simulink subsystem "PvtSubSys_PLAN_AP"  (R2020b)
settings: Solver=VariableStepAuto  StartTime=0.0  StopTime=10.0  RelTol=1e-3
undefined symbols (not defined in the file or in its folder): C_LongCtrl_0_Single, C_LongCtrl_0_Uint8, C_LongCtrl_Mph2Kph, magnitude, P_LongCtrl_accelTargAbsThrd, P_LongCtrl_AddVelAccelChange, P_LongCtrl_AddVelAccelThrd, P_LongCtrl_AddVelDistDesThrd, P_LongCtrl_AddVelEnable, P_LongCtrl_AddVelRefMsThrd, P_LongCtrl_ALaLowerChar, P_LongCtrl_ALaUpperCharEco, P_LongCtrl_ALaUpperCharNormal, P_LongCtrl_ALaUpperCharSport, P_LongCtrl_ALCAccLimitByDangerXAxis, P_LongCtrl_ALCAccLimitByDangerYAxis, P_LongCtrl_ALvAcceleLowerChar, P_LongCtrl_ALvAcceleUpperCharEco, P_LongCtrl_ALvAcceleUpperCharNormal, P_LongCtrl_ALvAcceleUpperCharSport, P_LongCtrl_CCaccelCCNeg2PosJerk, P_LongCtrl_CCaccelCCPosJerk, P_LongCtrl_CCaccelLowerIsLaneChange, P_LongCtrl_CCaccelMaxLCActive, P_LongCtrl_CCaccelMinECOAL, P_LongCtrl_CCaccelMinFastDecel, P_LongCtrl_CCaccelMinNoFastDecel, P_LongCtrl_CCaccelMinNormAL, P_LongCtrl_CCaccelMinSportAL, P_LongCtrl_CCaccelUpperCC, P_LongCtrl_CCaccelUpperCCSafeStop, P_LongCtrl_CCaMinNegAcceleLowerBand, P_LongCtrl_CCaMinNegAcceleUpperBand, P_LongCtrl_CCaMinPosAcceleLowerBand, P_LongCtrl_CCaMinPosAcceleUpperBand, P_LongCtrl_CCbECO, P_LongCtrl_CCbNorm, P_LongCtrl_CCbSport, P_LongCtrl_CCcoefESPSpd2IPSpd1, P_LongCtrl_CCcoefESPSpd2IPSpd2, P_LongCtrl_CCdecelCCJerk, P_LongCtrl_CCdecelCCJerkNegVLCInternalAcc, P_LongCtrl_CCfacNegAcceleLowerBand, P_LongCtrl_CCfacNegAcceleUpperBand, P_LongCtrl_CCfacPosAcceleLowerBand, P_LongCtrl_CCfacPosAcceleUpperBand, P_LongCtrl_CCkECO, P_LongCtrl_CCkNorm, P_LongCtrl_CCkSport, P_LongCtrl_CCLCIncSetSpdAdd, P_LongCtrl_CCLCIncSetSpdAddCntStartValue, P_LongCtrl_CCResumeDelayDeltaVel, P_LongCtrl_CCtAcceleTimeNeg, P_LongCtrl_CCtAcceleTimeNegCorrXAxis, P_LongCtrl_CCtAcceleTimeNegCorrYAxis, P_LongCtrl_CCtAcceleTimePos, P_LongCtrl_CCtAcceleTimePosCorrXAxis, P_LongCtrl_CCtAcceleTimePosCorrYAxis, P_LongCtrl_CCtStepVelPlan, P_LongCtrl_CCtTotVelPlan ... (+150)
libraries: simulink x62, TrueDurationTime x1
(part 4 of 7)

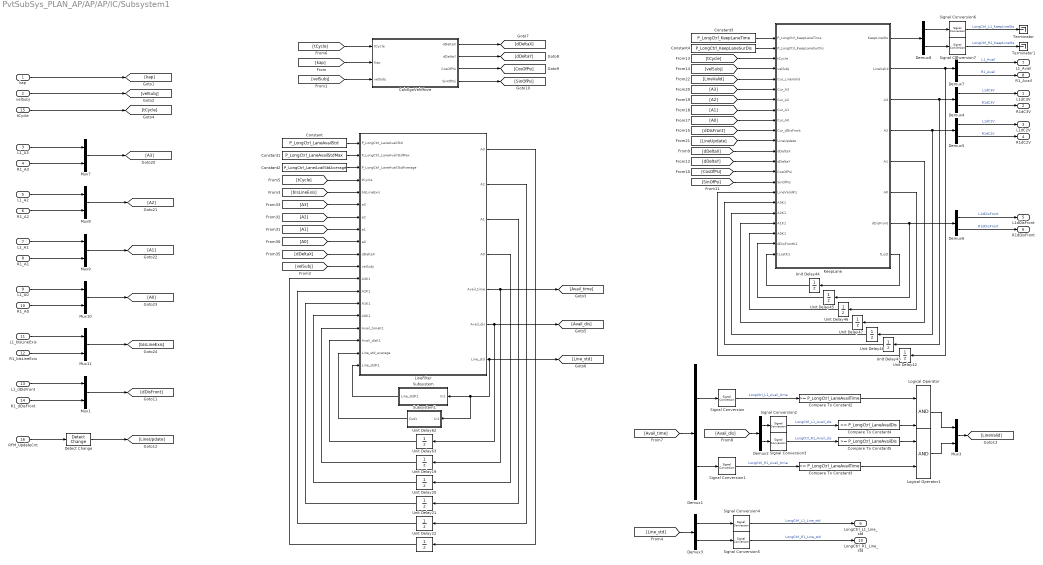
== system PvtSubSys_PLAN_AP/AP/AP/IC/Subsystem1 ==
  kap : Inport
  velSubj : Inport  Port=2
  L1_A3 : Inport  Port=3
  R1_A3 : Inport  Port=4
  L1_A2 : Inport  Port=5
  R1_A2 : Inport  Port=6
  L1_A1 : Inport  Port=7
  R1_A1 : Inport  Port=8
  L1_A0 : Inport  Port=9
  R1_A0 : Inport  Port=10
  L1_bIsLineExis : Inport  Port=11
  R1_bIsLineExis : Inport  Port=12
  L1_dDisFront : Inport  Port=13
  R1_dDisFront : Inport  Port=14
  tCycle : Inport  Port=15
  RFM_UpdateCnt : Inport  Port=16
  CalcEgoVehMove : MATLAB Function  TreatAsAtomicUnit=on
  Compare To Constant2 : simulink/Logic and Bit Operations/Compare To Constant  relop=>=  const=P_LongCtrl_LaneAvailTime  OutDataTypeStr=boolean
  Compare To Constant3 : simulink/Logic and Bit Operations/Compare To Constant  relop=>=  const=P_LongCtrl_LaneAvailTime  OutDataTypeStr=boolean
  Compare To Constant4 : simulink/Logic and Bit Operations/Compare To Constant  relop=>=  const=P_LongCtrl_LaneAvailDis  OutDataTypeStr=boolean
  Compare To Constant5 : simulink/Logic and Bit Operations/Compare To Constant  relop=>=  const=P_LongCtrl_LaneAvailDis  OutDataTypeStr=boolean
  Constant : Constant  Value=P_LongCtrl_LaneAvailStd
  Constant1 : Constant  Value=P_LongCtrl_LaneAvailStdMax
  Constant2 : Constant  Value=P_LongCtrl_LaneAvailStdAverage
  Constant3 : Constant  Value=P_LongCtrl_KeepLaneTime
  Constant4 : Constant  Value=P_LongCtrl_KeepLaneSurDis
  Demux{1..8} (8 alike) : Demux  Outputs=2
  Detect Change : simulink/Logic and Bit Operations/Detect Change  vinit=0  OutDataTypeStr=boolean
  KeepLane : MATLAB Function  TreatAsAtomicUnit=on
  LineFilter : MATLAB Function  TreatAsAtomicUnit=on
  Logical Operator : Logic  AllPortsSameDT=off  OutDataTypeStr=boolean
  Logical Operator1 : Logic  AllPortsSameDT=off  OutDataTypeStr=boolean
  Mux{1,3,7..11} (7 alike) : Mux  Inputs=2
  Signal Conversion{,1..7} (8 alike) : SignalConversion  OverrideOpt=off
  Subsystem : Subsystem
  Subsystem1 : Subsystem
  Terminator : Terminator
  Terminator1 : Terminator
  Unit Delay{19..22} (4 alike) : UnitDelay  InitialCondition=single(zeros(2,1))  SampleTime=-1  HasFrameUpgradeWarning=on
  Unit Delay42 : UnitDelay  InitialCondition=false  SampleTime=-1  HasFrameUpgradeWarning=on
  Unit Delay{43..48} (6 alike) : UnitDelay  InitialCondition=single(0)  SampleTime=-1  HasFrameUpgradeWarning=on
  Unit Delay62 : UnitDelay  InitialCondition=zeros(2,1)  SampleTime=-1  HasFrameUpgradeWarning=on
  Unit Delay63 : UnitDelay  InitialCondition=zeros(2,1)  SampleTime=-1  HasFrameUpgradeWarning=on
  L1dC3V : Outport
  R1dC3V : Outport  Port=2
  L1dC2V : Outport  Port=3
  R1dC2V : Outport  Port=4
  L1dDisFront : Outport  Port=5
  R1dDisFront : Outport  Port=6
  L1_Avail : Outport  Port=7
  R1_Avail : Outport  Port=8
  LongCtrl_L1_Line_std : Outport  Port=9
  LongCtrl_R1_Line_std : Outport  Port=10
  wires:
  Detect Change/1 -> [LineUpdate]
  [tCycle] -> CalcEgoVehMove/1(tCycle)
  [tCycle] -> LineFilter/4(tCycle)
  tCycle/1 -> [tCycle]
  [kap] -> CalcEgoVehMove/2(Kap)
  [velSubj] -> LineFilter/11(velSubj)
  Mux8/1 -> [A2]
  L1_bIsLineExis/1 -> Mux11/1
  L1_A1/1 -> Mux9/1
  kap/1 -> [kap]
  R1_bIsLineExis/1 -> Mux11/2
  Mux10/1 -> [A0]
  LineFilter/5(Avail_time) -> [Avail_time], Unit Delay63/1
  Mux7/1 -> [A3]
  L1_A2/1 -> Mux8/1
  Unit Delay19/1 -> LineFilter/15(A0K1)
  [A2] -> LineFilter/7(a2)
  Unit Delay22/1 -> LineFilter/12(A3K1)
  LineFilter/6(Avail_dis) -> [Avail_dis], Unit Delay62/1
  velSubj/1 -> [velSubj]
  [A1] -> LineFilter/8(a1)
  L1_A3/1 -> Mux7/1
  R1_A0/1 -> Mux10/2
  R1_A2/1 -> Mux8/2
  R1_A1/1 -> Mux9/2
  LineFilter/1(A3) -> Unit Delay22/1
  Unit Delay62/1 -> LineFilter/17(Avail_disK1)
  LineFilter/2(A2) -> Unit Delay21/1
  Mux9/1 -> [A1]
  [A0] -> LineFilter/9(a0)
  LineFilter/4(A0) -> Unit Delay19/1
  R1_A3/1 -> Mux7/2
  Mux11/1 -> [bIsLineExis]
  [bIsLineExis] -> LineFilter/5(bIsLineExis)
  [dDeltaX] -> LineFilter/10(dDeltaX)
  [velSubj] -> CalcEgoVehMove/3(velSubj)
  [A3] -> LineFilter/6(a3)
  LineFilter/3(A1) -> Unit Delay20/1
  Unit Delay20/1 -> LineFilter/14(A1K1)
  L1_A0/1 -> Mux10/1
  Unit Delay63/1 -> LineFilter/16(Avail_timeK1)
  Unit Delay21/1 -> LineFilter/13(A2K1)
  Compare To Constant3/1 -> Logical Operator1/2
  Logical Operator1/1 -> Mux3/2
  Signal Conversion1/1 -> Compare To Constant3/1  "LongCtrl_R1_Avail_time"
  Signal Conversion2/1 -> Compare To Constant4/1  "LongCtrl_L1_Avail_dis"
  Compare To Constant5/1 -> Logical Operator1/1
  Compare To Constant4/1 -> Logical Operator/2
  Logical Operator/1 -> Mux3/1
  Compare To Constant2/1 -> Logical Operator/1
  Signal Conversion3/1 -> Compare To Constant5/1  "LongCtrl_R1_Avail_dis"
  [Avail_time] -> Demux1/1
  Demux2/1 -> Signal Conversion2/1
  [Avail_dis] -> Demux2/1
  Demux2/2 -> Signal Conversion3/1
  Demux1/2 -> Signal Conversion1/1
  Demux1/1 -> Signal Conversion/1
  Signal Conversion/1 -> Compare To Constant2/1  "LongCtrl_L1_Avail_time"
  Constant/1 -> LineFilter/1(P_LongCtrl_LaneAvailStd)
  [Line_std] -> Demux3/1
  Signal Conversion5/1 -> LongCtrl_R1_Line_std/1  "LongCtrl_R1_Line_std"
  Signal Conversion4/1 -> LongCtrl_L1_Line_std/1  "LongCtrl_L1_Line_std"
  Demux3/1 -> Signal Conversion4/1
  Demux3/2 -> Signal Conversion5/1
  LineFilter/7(Line_std) -> [Line_std], Subsystem1/1(In1), Subsystem/1(In1)
  Subsystem/1(Line_stdK1) -> LineFilter/19(Line_stdK1)
  Subsystem1/1(Out1) -> LineFilter/18(Line_std_average)
  CalcEgoVehMove/1(dDeltaX) -> [dDeltaX]
  CalcEgoVehMove/2(dDeltaY) -> [dDeltaY]
  CalcEgoVehMove/4(SinOfPsi) -> [SinOfPsi]
  CalcEgoVehMove/3(CosOfPsi) -> [CosOfPsi]
  KeepLane/8(tLost) -> Unit Delay44/1
  Unit Delay42/1 -> KeepLane/16(LineValidK1)
  [CosOfPsi] -> KeepLane/14(CosOfPsi)
  [dDeltaY] -> KeepLane/13(dDeltaY)
  [dDeltaX] -> KeepLane/12(dDeltaX)
  Unit Delay43/1 -> KeepLane/17(A3K1)
  [SinOfPsi] -> KeepLane/15(SinOfPsi)
  Unit Delay48/1 -> KeepLane/18(A2K1)
  KeepLane/5(A1) -> Unit Delay47/1
  KeepLane/3(A3) -> Demux4/1, Unit Delay43/1
  Unit Delay46/1 -> KeepLane/20(A0K1)
  Unit Delay45/1 -> KeepLane/21(dDisFrontK1)
  Unit Delay44/1 -> KeepLane/22(tLostK1)
  KeepLane/2(LineValid) -> Demux7/1, Unit Delay42/1
  KeepLane/4(A2) -> Demux5/1, Unit Delay48/1
  KeepLane/6(A0) -> Unit Delay46/1
  Unit Delay47/1 -> KeepLane/19(A1K1)
  Mux1/1 -> [dDisFront]
  R1_dDisFront/1 -> Mux1/2
  L1_dDisFront/1 -> Mux1/1
  RFM_UpdateCnt/1 -> Detect Change/1
  Mux3/1 -> [LineValid]
  Constant1/1 -> LineFilter/2(P_LongCtrl_LaneAvailStdMax)
  Constant2/1 -> LineFilter/3(P_LongCtrl_LaneAvailStdAverage)
  [tCycle] -> KeepLane/3(tCycle)
  [velSubj] -> KeepLane/4(velSubj)
  [LineValid] -> KeepLane/5(Cur_LineValid)
  [A3] -> KeepLane/6(Cur_A3)
  [A2] -> KeepLane/7(Cur_A2)
  [A1] -> KeepLane/8(Cur_A1)
  [A0] -> KeepLane/9(Cur_A0)
  [dDisFront] -> KeepLane/10(Cur_dDisFront)
  [LineUpdate] -> KeepLane/11(LineUpdate)
  Constant3/1 -> KeepLane/1(P_LongCtrl_KeepLaneTime)
  Constant4/1 -> KeepLane/2(P_LongCtrl_KeepLaneSurDis)
  Demux4/1 -> L1dC3V/1  "L1dC3V"
  Demux4/2 -> R1dC3V/1  "R1dC3V"
  Demux5/2 -> R1dC2V/1  "R1dC2V"
  Demux5/1 -> L1dC2V/1  "L1dC2V"
  Demux6/1 -> L1dDisFront/1  "L1dDisFront"
  Demux6/2 -> R1dDisFront/1  "R1dDisFront"
  KeepLane/7(dDisFront) -> Unit Delay45/1, Demux6/1
  Demux7/2 -> R1_Avail/1  "R1_Avail"
  Demux7/1 -> L1_Avail/1  "L1_Avail"
  KeepLane/1(KeepLineSts) -> Demux8/1
  Demux8/1 -> Signal Conversion6/1
  Demux8/2 -> Signal Conversion7/1
  Signal Conversion6/1 -> Terminator/1  "LongCtrl_L1_KeepLineSts"
  Signal Conversion7/1 -> Terminator1/1  "LongCtrl_R1_KeepLineSts"

== system PvtSubSys_PLAN_AP/AP/AP/ORD/BandJerkCalc ==
  accelOffRamp : Inport
  Add : Sum
  Add1 : Sum  Inputs=+-
  Constant : Constant  Value=P_LongCtrl_ORDaccelDevUpperBand  OutDataTypeStr=single
  Constant1 : Constant  Value=P_LongCtrl_ORDaccelDevLowerBand  OutDataTypeStr=single
  Constant2 : Constant  Value=P_LongCtrl_ORDupperJerk  OutDataTypeStr=single
  Constant3 : Constant  Value=P_LongCtrl_ORDlowerJerk  OutDataTypeStr=single
  upperBandORD : Outport
  lowerBandORD : Outport  Port=2
  upperJerkORD : Outport  Port=3
  lowerJerkORD : Outport  Port=4
  wires:
  accelOffRamp/1 -> Add/1, Add1/1
  Constant/1 -> Add/2
  Constant1/1 -> Add1/2
  Add/1 -> upperBandORD/1  "upperBandORD"
  Add1/1 -> lowerBandORD/1  "lowerBandORD"
  Constant2/1 -> upperJerkORD/1  "upperJerkORD"
  Constant3/1 -> lowerJerkORD/1  "lowerJerkORD"

== system PvtSubSys_PLAN_AP/AP/AP/ORD/ORD/accelOffRampDistExceed ==
  distRamp2Cur : Inport  OutDataTypeStr=uint16  PortDimensions=1
  StartVel : Inport  Port=2  OutDataTypeStr=single  PortDimensions=1
  EndVel : Inport  Port=3  OutDataTypeStr=uint8  PortDimensions=1
  f : TriggerPort  TriggerType=function-call  VariantControl=(inherit)
      settings: CopyFcn=Stateflow.SLINSF.SimulinkMan.removeBlockPreDeleteFcn  PreDeleteFcn=Stateflow.SLINSF.SimulinkMan.unsafePredeleteFcn
  Add : Sum  Inputs=-+
  Constant : Constant  Value=2  OutDataTypeStr=single
  Constant2 : Constant  Value=10  OutDataTypeStr=single
  Constant3 : Constant  Value=3.6  OutDataTypeStr=single
  Constant4 : Constant  Value=3.6  OutDataTypeStr=single
  MinMax : MinMax  Function=max  Inputs=2
  Product : Product
  Product1 : Product  Inputs=*/
  Product3 : Product
  Product4 : Product
  Product5 : Product  Inputs=*/
  Product6 : Product  Inputs=*/
  accelOffRamp : Outport
  wires:
  Product4/1 -> Add/2
  Product3/1 -> Add/1
  Product6/1 -> Product4/1, Product4/2
  EndVel/1 -> Product6/1
  Constant4/1 -> Product6/2
  Constant3/1 -> Product5/2
  Product5/1 -> Product3/1, Product3/2
  StartVel/1 -> Product5/1
  distRamp2Cur/1 -> MinMax/1
  Constant/1 -> Product/2
  Add/1 -> Product1/1
  Product/1 -> Product1/2
  Product1/1 -> accelOffRamp/1  "accelOffRamp"
  Constant2/1 -> MinMax/2
  MinMax/1 -> Product/1

== system PvtSubSys_PLAN_AP/AP/AP/ORD/ORD/accelOffRampNegCalc ==
  velDelta : Inport  OutDataTypeStr=single  PortDimensions=1
  f : TriggerPort  TriggerType=function-call  VariantControl=(inherit)
      settings: CopyFcn=Stateflow.SLINSF.SimulinkMan.removeBlockPreDeleteFcn  PreDeleteFcn=Stateflow.SLINSF.SimulinkMan.unsafePredeleteFcn
  Constant : Constant  Value=P_LongCtrl_ORDtAcceleTimeNeg  OutDataTypeStr=single
  Product : Product  Inputs=*/
  accelOffRamp : Outport
  wires:
  velDelta/1 -> Product/1
  Constant/1 -> Product/2
  Product/1 -> accelOffRamp/1  "accelOffRamp"

== system PvtSubSys_PLAN_AP/AP/AP/ORD/ORD/accelOffRampPosCalc ==
  velDelta : Inport  OutDataTypeStr=single  PortDimensions=1
  f : TriggerPort  TriggerType=function-call  VariantControl=(inherit)
      settings: CopyFcn=Stateflow.SLINSF.SimulinkMan.removeBlockPreDeleteFcn  PreDeleteFcn=Stateflow.SLINSF.SimulinkMan.unsafePredeleteFcn
  Constant : Constant  Value=P_LongCtrl_ORDtAcceleTimePos  OutDataTypeStr=single
  Product : Product  Inputs=*/
  accelOffRamp : Outport
  wires:
  velDelta/1 -> Product/1
  Constant/1 -> Product/2
  Product/1 -> accelOffRamp/1  "accelOffRamp"

== system PvtSubSys_PLAN_AP/AP/AP/ORD/ORD/distDesOffRampCalc ==
  StartVel : Inport  OutDataTypeStr=single  PortDimensions=1
  EndVel : Inport  Port=2  OutDataTypeStr=uint8  PortDimensions=1
  accelOffRamp : Inport  Port=3  OutDataTypeStr=single  PortDimensions=1
  f : TriggerPort  TriggerType=function-call  VariantControl=(inherit)
      settings: CopyFcn=Stateflow.SLINSF.SimulinkMan.removeBlockPreDeleteFcn  PreDeleteFcn=Stateflow.SLINSF.SimulinkMan.unsafePredeleteFcn
  Abs : Abs
  Abs1 : Abs
  Add : Sum  Inputs=-+
  Constant : Constant  Value=2  OutDataTypeStr=single
  Constant3 : Constant  Value=3.6  OutDataTypeStr=single
  Constant4 : Constant  Value=3.6  OutDataTypeStr=single
  Product : Product  Inputs=*/
  Product1 : Product
  Product3 : Product
  Product4 : Product
  Product5 : Product  Inputs=*/
  Product6 : Product  Inputs=*/
  distDesOffRamp : Outport
  wires:
  Add/1 -> Abs1/1
  Constant4/1 -> Product6/2
  EndVel/1 -> Product6/1
  Product5/1 -> Product3/1, Product3/2
  StartVel/1 -> Product5/1
  Product6/1 -> Product4/1, Product4/2
  Product4/1 -> Add/2
  Constant3/1 -> Product5/2
  Product3/1 -> Add/1
  Abs1/1 -> Product/1
  accelOffRamp/1 -> Abs/1
  Constant/1 -> Product1/2
  Product1/1 -> Product/2
  Product/1 -> distDesOffRamp/1  "distDesOffRamp"
  Abs/1 -> Product1/1

== system PvtSubSys_PLAN_AP/AP/AP/ORD/ORD/velDeltaCalc ==
  velOffRampLimit : Inport  OutDataTypeStr=uint8  PortDimensions=1
  vehicleSpd : Inport  Port=2  OutDataTypeStr=single  PortDimensions=1
  f : TriggerPort  TriggerType=function-call  VariantControl=(inherit)
      settings: CopyFcn=Stateflow.SLINSF.SimulinkMan.removeBlockPreDeleteFcn  PreDeleteFcn=Stateflow.SLINSF.SimulinkMan.unsafePredeleteFcn
  Add : Sum  Inputs=+-
  Add1 : Sum
  Constant : Constant  Value=1.03  OutDataTypeStr=single
  Constant1 : Constant  Value=1.3  OutDataTypeStr=single
  Constant2 : Constant  Value=3.6  OutDataTypeStr=single
  Product : Product
  Product1 : Product  Inputs=*/
  velDelta : Outport
  IPKVel : Outport  Port=2
  wires:
  velOffRampLimit/1 -> Add/1
  vehicleSpd/1 -> Product/1
  Constant/1 -> Product/2
  Product/1 -> Add1/1
  Constant1/1 -> Add1/2
  Add1/1 -> Add/2, IPKVel/1
  Add/1 -> Product1/1
  Constant2/1 -> Product1/2
  Product1/1 -> velDelta/1  "velDelta"

== system PvtSubSys_PLAN_AP/AP/AP/SJ/BrakePreferJudge ==
  TargetExistP0 : Inport
  accelFollow : Inport  Port=2
  accelSubjPlanOpt : Inport  Port=3
  VlcInternalAccK1 : Inport  Port=4
  axvRoadSlopeMs2 : Inport  Port=5
  accelSubj : Inport  Port=6
  ttc : Inport  Port=7
  ACCModeSts : Inport  Port=8
  velSubj : Inport  Port=9
  HWASlowQuit : Inport  Port=10
  Compare To Constant : simulink/Logic and Bit Operations/Compare To Constant  relop===  const=1  OutDataTypeStr=boolean
  Compare To Constant1 : simulink/Logic and Bit Operations/Compare To Constant  relop=<  const=P_LongCtrl_SJaccelFollowThresEnableBrkPrefer  OutDataTypeStr=boolean
  Compare To Constant2 : simulink/Logic and Bit Operations/Compare To Constant  relop=<  const=P_LongCtrl_SJaccelSubjPlanOptThresEnableBrkPrefer  OutDataTypeStr=boolean
  Compare To Constant3 : simulink/Logic and Bit Operations/Compare To Constant  relop=<  const=P_LongCtrl_SJVlcInternalAccThresEnableBrkPrefer  OutDataTypeStr=boolean
  Compare To Constant4 : simulink/Logic and Bit Operations/Compare To Constant  relop=<  const=P_LongCtrl_SJaxvRoadSlopeThresEnableBrkPrefer  OutDataTypeStr=boolean
  Compare To Constant5 : simulink/Logic and Bit Operations/Compare To Constant  relop=>  const=P_LongCtrl_SJaccelSubjThresEnableBrkPrefer  OutDataTypeStr=boolean
  Compare To Constant6 : simulink/Logic and Bit Operations/Compare To Constant  relop=<  const=P_LongCtrl_SJttcThresEnableBrkPrefer  OutDataTypeStr=boolean
  Compare To Constant7 : simulink/Logic and Bit Operations/Compare To Constant  relop===  const=3  OutDataTypeStr=boolean
  Compare To Constant8 : simulink/Logic and Bit Operations/Compare To Constant  relop=>  const=P_LongCtrl_SJvelSubjThresEnableBrkPrefer  OutDataTypeStr=boolean
  Logical Operator : Logic  Inputs=9  AllPortsSameDT=off  OutDataTypeStr=boolean
  Logical Operator1 : Logic  Operator=OR  AllPortsSameDT=off  OutDataTypeStr=boolean
  MinMax : MinMax
  BrakePrefer : Outport
  wires:
  Logical Operator1/1 -> BrakePrefer/1  "BrakePrefer"
  TargetExistP0/1 -> Compare To Constant/1  "TargetExistP0"
  accelFollow/1 -> Compare To Constant1/1  "accelFollow"
  accelSubjPlanOpt/1 -> MinMax/1  "accelSubjPlanOpt"
  VlcInternalAccK1/1 -> Compare To Constant3/1  "VlcInternalAccK1"
  axvRoadSlopeMs2/1 -> Compare To Constant4/1  "axvRoadSlopeMs2"
  accelSubj/1 -> Compare To Constant5/1  "accelSubj"
  ttc/1 -> Compare To Constant6/1  "ttc"
  MinMax/1 -> Compare To Constant2/1
  ACCModeSts/1 -> Compare To Constant7/1  "ACCModeSts"
  Compare To Constant/1 -> Logical Operator/2
  Compare To Constant1/1 -> Logical Operator/3
  Compare To Constant2/1 -> Logical Operator/4
  Compare To Constant3/1 -> Logical Operator/5
  Compare To Constant4/1 -> Logical Operator/6
  Compare To Constant5/1 -> Logical Operator/7
  Compare To Constant7/1 -> Logical Operator/1
  Compare To Constant6/1 -> Logical Operator/8
  velSubj/1 -> Compare To Constant8/1  "velSubj"
  Compare To Constant8/1 -> Logical Operator/9
  Logical Operator/1 -> Logical Operator1/1  "BrakePrefer"
  HWASlowQuit/1 -> Logical Operator1/2  "HWASlowQuit"

== system PvtSubSys_PLAN_AP/AP/AP/SJ/DeceleToStop ==
  DriveOffConditonFulfilled : Inport
  TargetExistP0 : Inport  Port=2
  ACCModeSts : Inport  Port=3
  velSubj : Inport  Port=4
  velTargetRel : Inport  Port=5
  VlcInternalAcc : Inport  Port=6
  distTargRel : Inport  Port=7
  SafeStopActive : Inport  Port=8
  axvRoadSlopeMs2 : Inport  Port=9
  1-D Lookup Table : Lookup_n-D  NumberOfTableDimensions=1  BreakpointsForDimension1=P_LongCtrl_distThreDecToStopXAxis  Table=P_LongCtrl_distThreDecToStopYAxis  ExtrapMethod=Clip  InternalRulePriority=Speed  RndMeth=Simplest  InputSameDT=on
  DeceleToStop : Stateflow chart  TreatAsAtomicUnit=on
  DecleToStop : Outport
  wires:
  SafeStopActive/1 -> DeceleToStop/8(SafeStopActive)  "SafeStopActive"
  DriveOffConditonFulfilled/1 -> DeceleToStop/7(DriveOffConditonFulfilled)  "DriveOffConditonFulfilled"
  DeceleToStop/1(DecleToStop) -> DecleToStop/1  "DecleToStop"
  VlcInternalAcc/1 -> DeceleToStop/5(VlcInternalAcc)  "VlcInternalAcc"
  distTargRel/1 -> DeceleToStop/6(distTargRel)  "distTargRel"
  ACCModeSts/1 -> DeceleToStop/4(ACCModeSts)  "ACCModeSts"
  TargetExistP0/1 -> DeceleToStop/3(TargetExistP0)  "TargetExistP0"
  velTargetRel/1 -> DeceleToStop/2(velTargetRel)  "velTargetRel"
  velSubj/1 -> DeceleToStop/1(velSubj)  "velSubj"
  axvRoadSlopeMs2/1 -> 1-D Lookup Table/1  "axvRoadSlopeMs2"
  1-D Lookup Table/1 -> DeceleToStop/9(distThreDecToStop)

== system PvtSubSys_PLAN_AP/AP/AP/SJ/DisBar ==
  distTargRel : Inport
  DesireDistanceChar : Inport  Port=2
  timeGapSet : Inport  Port=3
  ACCSts_ACCModeSts : Inport  Port=4
  P0_Exist : Inport  Port=5
  distTargRelP2 : Inport  Port=6
  distTargRelP3 : Inport  Port=7
  P2_Exist : Inport  Port=8
  P3_Exist : Inport  Port=9
  ACC_DisplayBar1 : Subsystem  TreatAsAtomicUnit=on
  Constant18 : Constant  Value=[0.6,0.75,0.9;0.58,0.68,0.77;0.41,0.55,0.63;0.38,0.44,0.49]  OutDataTypeStr=single
  Demux : Demux  Outputs=3
  Mux2 : Mux  Inputs=3
  Mux3 : Mux  Inputs=3
  Signal Conversion : SignalConversion  OverrideOpt=off
  Signal Conversion1 : SignalConversion  OverrideOpt=off
  Signal Conversion2 : SignalConversion  OverrideOpt=off
  ACC_TgtObjBarDisp : Outport  OutDataTypeStr=uint8
  ACC_LeTgtObjBarDisp : Outport  Port=2
  ACC_RiTgtObjBarDisp : Outport  Port=3
  wires:
  Signal Conversion2/1 -> ACC_RiTgtObjBarDisp/1
  Signal Conversion1/1 -> ACC_LeTgtObjBarDisp/1
  Signal Conversion/1 -> ACC_TgtObjBarDisp/1
  P3_Exist/1 -> Mux3/3
  P0_Exist/1 -> Mux3/1
  distTargRelP2/1 -> Mux2/2
  Constant18/1 -> ACC_DisplayBar1/5(Scale)
  distTargRelP3/1 -> Mux2/3
  Mux2/1 -> ACC_DisplayBar1/4(TargetRange)
  P2_Exist/1 -> Mux3/2
  Mux3/1 -> ACC_DisplayBar1/6(TargetExist)
  ACC_DisplayBar1/1(Signal_ACC_TgtObjBarDisp) -> Demux/1  "ACC_TgtObjBarDisp"
  Demux/2 -> Signal Conversion1/1  "ACC_LeTgtObjBarDisp"
  Demux/1 -> Signal Conversion/1  "ACC_TgtObjBarDisp"
  Demux/3 -> Signal Conversion2/1  "ACC_RiTgtObjBarDisp"
  distTargRel/1 -> Mux2/1  "distTargRel"
  timeGapSet/1 -> ACC_DisplayBar1/1(TimeGap)  "timeGapSet"
  DesireDistanceChar/1 -> ACC_DisplayBar1/2(DesireDistance)
  ACCSts_ACCModeSts/1 -> ACC_DisplayBar1/3(ACCmode)

== system PvtSubSys_PLAN_AP/AP/AP/SJ/DriverOffConditionFulfilled ==
  TargetExistP0 : Inport
  velTargetRel : Inport  Port=2
  VelSet : Inport  Port=3  OutDataTypeStr=single
  distDesCur : Inport  Port=4
  velSubj : Inport  Port=5
  distTargRel : Inport  Port=6
  safeStopActive : Inport  Port=7
  ACCModeSts : Inport  Port=8
  ObjTypeP0 : Inport  Port=9
  Compare To Constant : simulink/Logic and Bit Operations/Compare To Constant  relop===  const=0  OutDataTypeStr=boolean
  Compare To Constant1 : simulink/Logic and Bit Operations/Compare To Constant  relop=>  const=0  OutDataTypeStr=boolean
  Constant : Constant  Value=0  OutDataTypeStr=uint8
  DriveOff_Judge : Stateflow chart  TreatAsAtomicUnit=on
  Gain : Gain  Gain=1/3.6
  Switch : Switch  Criteria=u2 > Threshold
  DriveOffConditonFulfilled : Outport  OutDataTypeStr=boolean
  wires:
  ObjTypeP0/1 -> DriveOff_Judge/8(ObjTypeP0)
  safeStopActive/1 -> Compare To Constant/1
  Compare To Constant/1 -> Switch/2
  velSubj/1 -> DriveOff_Judge/1(velSubj)  "velSubj"
  VelSet/1 -> Gain/1  "VelSet"
  velTargetRel/1 -> DriveOff_Judge/4(velTargRel)  "velTargetRel"
  distTargRel/1 -> DriveOff_Judge/5(distTargRel)  "distTargRel"
  TargetExistP0/1 -> DriveOff_Judge/6(targetExist)  "TargetExistP0"
  Constant/1 -> Switch/3
  Gain/1 -> DriveOff_Judge/3(velSet)
  Compare To Constant1/1 -> DriveOffConditonFulfilled/1
  ACCModeSts/1 -> DriveOff_Judge/7(ACCModeSts)  "ACCModeSts"
  DriveOff_Judge/1(DriveOffConditonFulfilled) -> Switch/1
  Switch/1 -> Compare To Constant1/1  "DriveOffConditonFulfilled"
  distDesCur/1 -> DriveOff_Judge/2(dDesired)  "distDesCur"

== system PvtSubSys_PLAN_AP/AP/AP/SJ/TakeOver ==
  accelFollow : Inport
  ACCModeSts : Inport  Port=2
  distTargetRel : Inport  Port=3
  velSubj : Inport  Port=4
  targetExistP0 : Inport  Port=5
  distRelPlanMin : Inport  Port=6
  distRelDesDistRelPlanNumMin : Inport  Port=7
  velTargetRel : Inport  Port=8
  tCycle : Inport  Port=9
  Chart : Stateflow chart  TreatAsAtomicUnit=on
      settings: PortSchema="{\"entries\":[{\"content\":{\"sides\":[{\"content\":{\"connectorIds\":[\"In1\",\"In2\",\"In3\"]},\"type\":\"ConnectorPlacement.EquallySpacedRectSide\",\"uuid\":\"a9be611c-1302-4d01-95c8-aa310eaae015\"},{\"content\":{\"connectorIds\":[\"Out2\",\"Out1\"],\"side\":\"RIGHT\"},\"type\":\"ConnectorPlacement.EquallySpacedRectSide\",\"uuid\":\"1ce4f311-da37-41d3-8dab-86903ba1c2a6\"},{\"content\":{\"connectorIds\":[],\"side\":\"TOP\"},\"type\":\"ConnectorPlacement.EquallySpacedRectSide\",\"uuid\":\"6f48286d-1440-4f3e-bf88-8b89e91ed982\"},{\"content\":{\"connectorIds\":[],\"side\":\"HIDDEN\"},\"type\":\"ConnectorPlacement.EquallySpacedRectSide\",\"uuid\":\"bdda7e3f-a505-4bee-9100-0395b80b4afd\"}]},\"type\":\"ConnectorPlacement.EquallySpacedConnector\",\"uuid\":\"e8fe679d-9fc6-4d49-831a-9b3ad6242aaa\"}],\"packageUris\":[\"http://schema.mathworks.com/mf0/Connector/R2020b\"],\"version\":\"1.0\"}"
  Constant : Constant  Value=P_LongCtrl_WaitTime
  Divide : Product  Inputs=*/
  Gap : Subsystem
  TakeOver : Stateflow chart  TreatAsAtomicUnit=on
  Terminator : Terminator
  tor : Outport
  wires:
  ACCModeSts/1 -> TakeOver/1(ACCModeSts)
  accelFollow/1 -> TakeOver/3(accelFollow)
  distTargetRel/1 -> Gap/1(distTargetRel)
  velSubj/1 -> Gap/2(velSubj)
  Gap/1(gap) -> TakeOver/2(gap)
  targetExistP0/1 -> TakeOver/4(targetExistP0)
  distRelPlanMin/1 -> Chart/2(distRelPlanMin)
  distRelDesDistRelPlanNumMin/1 -> Chart/3(distRelDesDistRelPlanNumMin)
  velTargetRel/1 -> TakeOver/5(velTargetRel)
  TakeOver/1(tor) -> tor/1
  Divide/1 -> Chart/1(WaitSteps)
  Constant/1 -> Divide/1
  tCycle/1 -> Divide/2
  Chart/1(Cnt) -> Terminator/1
  Chart/2(TorCtrlReq) -> TakeOver/6(TorCtrlReq)

== system PvtSubSys_PLAN_AP/AP/AP/FollowCtrl/AccelTargFilter/accelTargAbsFilter/tFiltP0Calc ==
  diffAccelCur2K1P0 : Inport  OutDataTypeStr=single  PortDimensions=1
  f : TriggerPort  TriggerType=function-call  VariantControl=Variant
      settings: CopyFcn=Stateflow.SLINSF.SimulinkMan.removeBlockPreDeleteFcn  PreDeleteFcn=Stateflow.SLINSF.SimulinkMan.unsafePredeleteFcn
  1-D Lookup Table : Lookup_n-D  NumberOfTableDimensions=1  BreakpointsForDimension1=P_LongCtrl_FollowTFiltP0XAxis  Table=P_LongCtrl_FollowTFiltP0YAxis  ExtrapMethod=Clip  InternalRulePriority=Speed  RndMeth=Simplest  InputSameDT=on
  tFiltP0 : Outport
  wires:
  1-D Lookup Table/1 -> tFiltP0/1  "tFiltP0"
  diffAccelCur2K1P0/1 -> 1-D Lookup Table/1

== system PvtSubSys_PLAN_AP/AP/AP/FollowCtrl/DecelToStopCtrl/DecelToStopCtrl ==
  note: when runtime is 50ms,this value is -0.025.
  note: when runtime is 20ms,this value is -0.01.
  FollowAccelMPC : Inport
  accelTargAbs : Inport  Port=2
  distTargRel : Inport  Port=3
  velSubj : Inport  Port=4
  distDesCur : Inport  Port=5
  velTargAbs : Inport  Port=6
  ACCModeSts : Inport  Port=7  OutDataTypeStr=uint8
  DrvOFF_Req : Inport  Port=8
  axvRoadSlopeMs2 : Inport  Port=9
  ObjMovingStateP0 : Inport  Port=10
  DecelToStopCtrl : Stateflow chart  TreatAsAtomicUnit=on
      settings: PortSchema="{\"entries\":[{\"content\":{\"sides\":[{\"content\":{\"connectorIds\":[\"In1\",\"In2\",\"In3\",\"In4\",\"In5\",\"In6\",\"In7\",\"In8\",\"In9\",\"In10\",\"In11\",\"In12\",\"In13\",\"In14\",\"In15\",\"In16\",\"In17\",\"In18\",\"In19\",\"In20\",\"In22\",\"In23\",\"In24\",\"In25\",\"In26\",\"In21\"]},\"type\":\"ConnectorPlacement.EquallySpacedRectSide\",\"uuid\":\"c20511a8-015c-4635-8210-b9eed3497188\"},{\"content\":{\"connectorIds\":[\"Out1\",\"Out2\"],\"side\":\"RIGHT\"},\"type\":\"ConnectorPlacement.EquallySpacedRectSide\",\"uuid\":\"1a046c23-c67c-4e6f-902f-f121eb708ec4\"},{\"content\":{\"connectorIds\":[],\"side\":\"TOP\"},\"type\":\"ConnectorPlacement.EquallySpacedRectSide\",\"uuid\":\"c73ac045-3121-4509-a6aa-8453b68f107e\"},{\"content\":{\"connectorIds\":[],\"side\":\"HIDDEN\"},\"type\":\"ConnectorPlacement.EquallySpacedRectSide\",\"uuid\":\"793d462e-a4a7-4165-a400-0e9fce0ddd3d\"}]},\"type\":\"ConnectorPlacement.EquallySpacedConnector\",\"uuid\":\"1cf22de0-f5b0-4ce2-b122-91219d3d6299\"}],\"packageUris\":[\"http://schema.mathworks.com/mf0/Connector/R2020b\"],\"version\":\"1.0\"}"
  P_LongCtrl_AddVelAccelChange : Constant  Value=P_LongCtrl_AddVelAccelChange
  P_LongCtrl_AddVelAccelThrd : Constant  Value=P_LongCtrl_AddVelAccelThrd
  P_LongCtrl_AddVelDistDesThrd : Constant  Value=P_LongCtrl_AddVelDistDesThrd
  P_LongCtrl_AddVelEnable : Constant  Value=P_LongCtrl_AddVelEnable
  P_LongCtrl_AddVelRefMsThrd : Constant  Value=P_LongCtrl_AddVelRefMsThrd
  P_LongCtrl_FollowaccelStopMax : Constant  Value=P_LongCtrl_FollowaccelStopMax  OutDataTypeStr=single
  P_LongCtrl_FollowaccelTargThresEnableStop : Constant  Value=P_LongCtrl_FollowaccelTargThresEnableStop  OutDataTypeStr=single
  P_LongCtrl_FollowaccelTargThresForceStop : Constant  Value=P_LongCtrl_FollowaccelTargThresForceStop  OutDataTypeStr=single
  P_LongCtrl_FollowdistThresEnableStop : Constant  Value=P_LongCtrl_FollowdistThresEnableStop  OutDataTypeStr=single
  P_LongCtrl_FollowvelSubjThresEnableStop : Constant  Value=P_LongCtrl_FollowvelSubjThresEnableStop  OutDataTypeStr=single
  P_LongCtrl_FollowvelTarAbsThresForceStop : Constant  Value=P_LongCtrl_FollowvelTarAbsThresForceStop  OutDataTypeStr=single
  P_LongCtrl_jerkForceStop : Constant  Commented=on  Value=-0.025  OutDataTypeStr=single
  P_LongCtrl_jerkForceStop1 : Constant  Commented=on  Value=-0.01  OutDataTypeStr=single
  P_LongCtrl_velSubjThresEnableStopAdd : Subsystem
  Subsystem : Subsystem
  FollowAccel : Outport
  ForceStop : Outport  Port=2
  wires:
  P_LongCtrl_AddVelAccelChange/1 -> DecelToStopCtrl/26(P_LongCtrl_AddVelAccelChange)
  P_LongCtrl_AddVelEnable/1 -> DecelToStopCtrl/25(P_LongCtrl_AddVelEnable)
  P_LongCtrl_AddVelRefMsThrd/1 -> DecelToStopCtrl/24(P_LongCtrl_AddVelRefMsThrd)
  P_LongCtrl_AddVelDistDesThrd/1 -> DecelToStopCtrl/23(P_LongCtrl_AddVelDistDesThrd)
  P_LongCtrl_AddVelAccelThrd/1 -> DecelToStopCtrl/22(P_LongCtrl_AddVelAccelThrd)
  ObjMovingStateP0/1 -> DecelToStopCtrl/21(ObjMovingStateP0)
  DrvOFF_Req/1 -> DecelToStopCtrl/7(DrvOFF_Req)  "DrvOFF_Req"
  P_LongCtrl_FollowvelTarAbsThresForceStop/1 -> DecelToStopCtrl/20(P_LongCtrl_velTarAbsThresForceStop)
  velTargAbs/1 -> DecelToStopCtrl/5(velTargAbs)
  ACCModeSts/1 -> DecelToStopCtrl/6(ACCModeSts)
  P_LongCtrl_FollowaccelTargThresForceStop/1 -> DecelToStopCtrl/19(P_LongCtrl_accelTargThresForceStop)
  distDesCur/1 -> DecelToStopCtrl/4(distDesCur)
  accelTargAbs/1 -> DecelToStopCtrl/1(accelTargAbs)
  distTargRel/1 -> DecelToStopCtrl/8(distTargRel), P_LongCtrl_velSubjThresEnableStopAdd/1(distTargRel)
  velSubj/1 -> DecelToStopCtrl/2(velSubj)
  FollowAccelMPC/1 -> DecelToStopCtrl/3(FollowAccelDes)
  P_LongCtrl_FollowdistThresEnableStop/1 -> DecelToStopCtrl/15(P_LongCtrl_distThresEnableStop)
  P_LongCtrl_FollowvelSubjThresEnableStop/1 -> DecelToStopCtrl/16(P_LongCtrl_velSubjThresEnableStop)
  P_LongCtrl_FollowaccelTargThresEnableStop/1 -> DecelToStopCtrl/17(P_LongCtrl_accelTargThresEnableStop)
  P_LongCtrl_FollowaccelStopMax/1 -> DecelToStopCtrl/18(P_LongCtrl_accelStopMax)
  DecelToStopCtrl/1(FollowAccel) -> FollowAccel/1
  DecelToStopCtrl/2(ForceStop) -> ForceStop/1  "ForceStop"
  P_LongCtrl_velSubjThresEnableStopAdd/2(velSubjThresEnableStopAdd) -> DecelToStopCtrl/10(velSubjThresEnableStopAdd)
  P_LongCtrl_velSubjThresEnableStopAdd/1(accelFollowDesThresEnableStop) -> DecelToStopCtrl/9(accelFollowDesThresEnableStop)
  axvRoadSlopeMs2/1 -> Subsystem/1(axvRoadSlopeMs2)
  Subsystem/1(velSubjThresForceStop) -> DecelToStopCtrl/12(velSubjThresForceStop), P_LongCtrl_velSubjThresEnableStopAdd/2(velSubjThresForceStop)
  Subsystem/2(jerkForceStop) -> DecelToStopCtrl/13(jerkForceStop)
  Subsystem/3(accelForceMin) -> DecelToStopCtrl/14(accelForceMin)
  P_LongCtrl_velSubjThresEnableStopAdd/3(velSubjThresForceStopStationaryTarget) -> DecelToStopCtrl/11(velSubjThresForceStopStationaryTarget)

== system PvtSubSys_PLAN_AP/AP/AP/FollowCtrl/FollowBandJerkCalc/AccelFollowAfterJerk ==
  accelFollow : Inport
  VlcInternalAccK1 : Inport  Port=2
  tCycle : Inport  Port=3
  lowerJerkFollow : Inport  Port=4
  " upperJerkFollow" : Inport  Port=5
  Add1 : Sum
  Add2 : Sum
  MinMax : MinMax  Function=max  Inputs=2
  MinMax1 : MinMax  Inputs=2  OutDataTypeStr=single
  Product : Product
  Product1 : Product
  accelFollowAfterJerk : Outport  OutDataTypeStr=single
  wires:
  accelFollow/1 -> MinMax/1
  Add2/1 -> MinMax/2
  lowerJerkFollow/1 -> Product/1
  Product/1 -> Add2/2
  tCycle/1 -> Product1/1, Product/2
  VlcInternalAccK1/1 -> [VlcInternalAccK1], Add2/1
  " upperJerkFollow"/1 -> Product1/2
  [VlcInternalAccK1] -> Add1/1
  Product1/1 -> Add1/2
  MinMax/1 -> MinMax1/1
  Add1/1 -> MinMax1/2
  MinMax1/1 -> accelFollowAfterJerk/1  "LongCtrl_accelFollowAfterJerk"

== system PvtSubSys_PLAN_AP/AP/AP/FollowCtrl/FollowBandJerkCalc/AccelFollowJerkCalc ==
  VlcInternalAccK1 : Inport
  FollowAccele : Inport  Port=2
  velSubj : Inport  Port=3
  1-D Lookup Table : Lookup_n-D  NumberOfTableDimensions=1  BreakpointsForDimension1=P_LongCtrl_FollowAccelCharNegVlcAcc2CoefEnlargeAccelJerkXAxis  Table=P_LongCtrl_FollowCoefCharCoefEnlargeAccelJerkYAxis  ExtrapMethod=Clip  InternalRulePriority=Speed  RndMeth=Simplest  InputSameDT=on
  1-D Lookup Table1 : Lookup_n-D  NumberOfTableDimensions=1  BreakpointsForDimension1=P_LongCtrl_FollowVelCharAccelJerkXAxis  Table=P_LongCtrl_FollowJerkCharAccelJerkYAxis  ExtrapMethod=Clip  InternalRulePriority=Speed  RndMeth=Simplest  InputSameDT=on
  Compare To Zero : simulink/Logic and Bit Operations/Compare To Zero  relop=<=  OutDataTypeStr=boolean
  Constant : Constant  Value=P_LongCtrl_FollowAccelJerkNegFollowAccel  OutDataTypeStr=single
  Product : Product
  Switch : Switch  Criteria=u2 > Threshold
  accelFollowJerk : Outport
  wires:
  Compare To Zero/1 -> Switch/2
  Switch/1 -> Product/2
  1-D Lookup Table/1 -> Product/1
  1-D Lookup Table1/1 -> Switch/3
  Constant/1 -> Switch/1
  FollowAccele/1 -> Compare To Zero/1
  Product/1 -> accelFollowJerk/1
  VlcInternalAccK1/1 -> 1-D Lookup Table/1
  velSubj/1 -> 1-D Lookup Table1/1

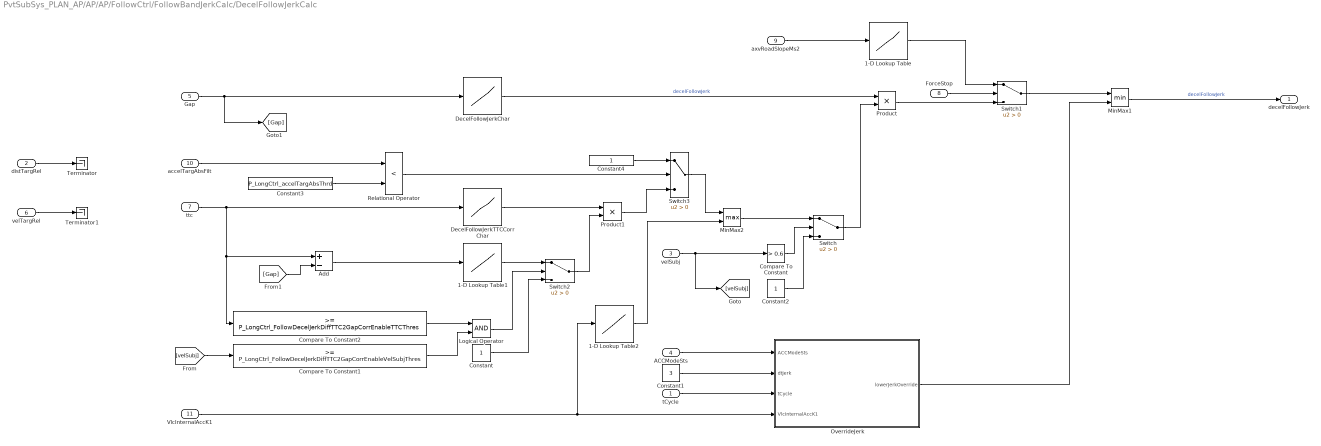
== system PvtSubSys_PLAN_AP/AP/AP/FollowCtrl/FollowBandJerkCalc/DecelFollowJerkCalc ==
  tCycle : Inport
  distTargRel : Inport  Port=2
  velSubj : Inport  Port=3
  ACCModeSts : Inport  Port=4  OutDataTypeStr=uint8
  Gap : Inport  Port=5
  velTargRel : Inport  Port=6
  ttc : Inport  Port=7
  ForceStop : Inport  Port=8
  axvRoadSlopeMs2 : Inport  Port=9
  accelTargAbsFilt : Inport  Port=10
  VlcInternalAccK1 : Inport  Port=11
  1-D Lookup Table : Lookup_n-D  NumberOfTableDimensions=1  BreakpointsForDimension1=P_LongCtrl_FollowDecelJerkForceSlopeXAxis  Table=P_LongCtrl_FollowDecelJerkForceSlopeYAxis  ExtrapMethod=Clip  InternalRulePriority=Speed  RndMeth=Simplest  InputSameDT=on
  1-D Lookup Table1 : Lookup_n-D  NumberOfTableDimensions=1  BreakpointsForDimension1=P_LongCtrl_FollowDecelJerkDiffTTC2GapCorrXAxis  Table=P_LongCtrl_FollowDecelJerkDiffTTC2GapCorrYAxis  ExtrapMethod=Clip  InternalRulePriority=Speed  RndMeth=Simplest  InputSameDT=on
  1-D Lookup Table2 : Lookup_n-D  NumberOfTableDimensions=1  BreakpointsForDimension1=[0 0.5]  Table=[0 1]  ExtrapMethod=Clip  InternalRulePriority=Speed  RndMeth=Simplest  InputSameDT=on
  Add : Sum  Inputs=+-
  Compare To Constant : simulink/Logic and Bit Operations/Compare To Constant  relop=>  const=0.6  OutDataTypeStr=boolean
  Compare To Constant1 : simulink/Logic and Bit Operations/Compare To Constant  relop=>=  const=P_LongCtrl_FollowDecelJerkDiffTTC2GapCorrEnableVelSubjThres  OutDataTypeStr=boolean
  Compare To Constant2 : simulink/Logic and Bit Operations/Compare To Constant  relop=>=  const=P_LongCtrl_FollowDecelJerkDiffTTC2GapCorrEnableTTCThres  OutDataTypeStr=boolean
  Constant : Constant  OutDataTypeStr=single
  Constant1 : Constant  Value=3  OutDataTypeStr=single
  Constant2 : Constant  OutDataTypeStr=single
  Constant3 : Constant  Value=P_LongCtrl_accelTargAbsThrd  OutDataTypeStr=single
  Constant4 : Constant  OutDataTypeStr=single
  DecelFollowJerkChar : Lookup_n-D  NumberOfTableDimensions=1  BreakpointsForDimension1=P_LongCtrl_FollowdecelJerkCharXAxis  Table=P_LongCtrl_FollowdecelJerkCharYAxis  ExtrapMethod=Clip  InternalRulePriority=Speed  RndMeth=Simplest  InputSameDT=on
  DecelFollowJerkTTCCorrChar : Lookup_n-D  NumberOfTableDimensions=1  BreakpointsForDimension1=P_LongCtrl_FollowttcCorrDecelJerkXAxis  Table=P_LongCtrl_FollowttcCorrDecelJerkYAxis  ExtrapMethod=Clip  InternalRulePriority=Speed  RndMeth=Simplest  InputSameDT=on
  Logical Operator : Logic  AllPortsSameDT=off  OutDataTypeStr=boolean
  MinMax1 : MinMax  Inputs=2
  MinMax2 : MinMax  Function=max  Inputs=2
  OverrideJerk : Stateflow chart  TreatAsAtomicUnit=on
  Product : Product
  Product1 : Product
  Relational Operator : RelationalOperator  Operator=<  OutDataTypeStr=boolean  RndMeth=Simplest
  Switch{,1..3} (4 alike) : Switch  Criteria=u2 > Threshold
  Terminator : Terminator
  Terminator1 : Terminator
  decelFollowJerk : Outport
  wires:
  Constant4/1 -> Switch3/1
  Switch3/1 -> MinMax2/1
  Relational Operator/1 -> Switch3/2
  Constant3/1 -> Relational Operator/2
  accelTargAbsFilt/1 -> Relational Operator/1
  ttc/1 -> DecelFollowJerkTTCCorrChar/1, Add/1, Compare To Constant2/1
  velTargRel/1 -> Terminator1/1
  distTargRel/1 -> Terminator/1
  Switch/1 -> Product/2
  Constant2/1 -> Switch/3
  Compare To Constant/1 -> Switch/2
  Switch1/1 -> MinMax1/1
  MinMax2/1 -> Switch/1
  1-D Lookup Table2/1 -> MinMax2/2
  Product1/1 -> Switch3/3
  DecelFollowJerkChar/1 -> Product/1  "decelFollowJerk"
  VlcInternalAccK1/1 -> 1-D Lookup Table2/1, OverrideJerk/4(VlcInternalAccK1)
  OverrideJerk/1(lowerJerkOverride) -> MinMax1/2
  tCycle/1 -> OverrideJerk/3(tCycle)
  Constant1/1 -> OverrideJerk/2(dtJerk)
  ACCModeSts/1 -> OverrideJerk/1(ACCModeSts)
  MinMax1/1 -> decelFollowJerk/1  "decelFollowJerk"
  Gap/1 -> DecelFollowJerkChar/1, [Gap]
  velSubj/1 -> [velSubj], Compare To Constant/1
  ForceStop/1 -> Switch1/2
  Product/1 -> Switch1/3
  1-D Lookup Table/1 -> Switch1/1
  axvRoadSlopeMs2/1 -> 1-D Lookup Table/1
  [velSubj] -> Compare To Constant1/1
  Add/1 -> 1-D Lookup Table1/1
  Compare To Constant2/1 -> Logical Operator/1
  Compare To Constant1/1 -> Logical Operator/2
  Logical Operator/1 -> Switch2/2
  [Gap] -> Add/2
  1-D Lookup Table1/1 -> Switch2/1
  Constant/1 -> Switch2/3
  DecelFollowJerkTTCCorrChar/1 -> Product1/1
  Switch2/1 -> Product1/2

== system PvtSubSys_PLAN_AP/AP/AP/FollowCtrl/FollowBandJerkCalc/LP ==
  accelFollow : Inport
  IDP0 : Inport  Port=2
  Add : Sum  Inputs=+-
  Add1 : Sum
  Compare To Constant : simulink/Logic and Bit Operations/Compare To Constant  relop===  const=0  OutDataTypeStr=boolean
  Constant : Constant  Value=0.3  OutDataTypeStr=single
  Logical Operator : Logic  Operator=OR  AllPortsSameDT=off  OutDataTypeStr=boolean
  Product1 : Product
  Relational Operator : RelationalOperator  Operator=~=  OutDataTypeStr=boolean  RndMeth=Simplest
  Switch : Switch  Criteria=u2 ~= 0
  Unit Delay : UnitDelay  SampleTime=-1  HasFrameUpgradeWarning=on
  Unit Delay1 : UnitDelay  SampleTime=-1  HasFrameUpgradeWarning=on
  accelFollowFilt : Outport
  wires:
  accelFollow/1 -> Switch/1, Add/1  "accelFollow"
  Product1/1 -> Add1/1
  Constant/1 -> Product1/1
  Add/1 -> Product1/2
  Unit Delay/1 -> Add/2, Add1/2
  Switch/1 -> accelFollowFilt/1, Unit Delay/1  "LongCtrl_accelFollowFilt"
  IDP0/1 -> Relational Operator/2, Unit Delay1/1
  Unit Delay1/1 -> Relational Operator/1, Compare To Constant/1
  Compare To Constant/1 -> Logical Operator/1
  Relational Operator/1 -> Logical Operator/2
  Logical Operator/1 -> Switch/2
  Add1/1 -> Switch/3

== system PvtSubSys_PLAN_AP/AP/AP/FollowCtrl/FollowBandJerkCalc/Subsystem ==
  accelFollowFilt : Inport  OutDataTypeStr=single
  Add : Sum
  Add1 : Sum  Inputs=+-
  Constant : Constant  Value=0.2  OutDataTypeStr=single
  Constant1 : Constant  Value=0.2  OutDataTypeStr=single
  upperBandFollow : Outport
  lowerBandFollow : Outport  Port=2
  wires:
  Add1/1 -> lowerBandFollow/1  "lowerBandFollow"
  Constant/1 -> Add/1  "FollowAcceleUpperBand"
  Constant1/1 -> Add1/2  "FollowAcceleLowerBand"
  accelFollowFilt/1 -> Add1/1, Add/2
  Add/1 -> upperBandFollow/1  "upperBandFollow"

== system PvtSubSys_PLAN_AP/AP/AP/FollowCtrl/PlausibilityCheck/StandstillOverrideAccelLimit ==
  followAccel_Plau : Inport
  standstillOverrideCondition : Inport  Port=2  OutDataTypeStr=boolean
  coefStandstillOverride : Inport  Port=3
  quickDecel : Inport  Port=4
  Constant : Constant  Value=-0.2  OutDataTypeStr=single
  Constant1 : Constant  Value=10  OutDataTypeStr=single
  Constant2 : Constant  Value=-10  OutDataTypeStr=single
  Constant3 : Constant  Value=10  OutDataTypeStr=single
  Constant4 : Constant  Value=P_LongCtrl_FollowQuickDecelAccelDesMax
  MinMax : MinMax  Inputs=2
  MinMax1 : MinMax  Function=max  Inputs=2
  MinMax2 : MinMax  Inputs=2
  Product : Product
  Switch : Switch  Criteria=u2 > Threshold
  Switch1 : Switch  Criteria=u2 > Threshold
  followAcceleStandstillOverride : Outport
  wires:
  standstillOverrideCondition/1 -> Switch/2
  MinMax1/1 -> followAcceleStandstillOverride/1
  Constant/1 -> Switch/1
  Constant1/1 -> Switch/3
  Switch/1 -> MinMax/1
  followAccel_Plau/1 -> MinMax/2
  MinMax2/1 -> Product/1
  coefStandstillOverride/1 -> Product/2
  Product/1 -> MinMax1/1
  Constant2/1 -> MinMax1/2
  quickDecel/1 -> Switch1/2
  MinMax/1 -> MinMax2/1
  Switch1/1 -> MinMax2/2
  Constant3/1 -> Switch1/3
  Constant4/1 -> Switch1/1

== system PvtSubSys_PLAN_AP/AP/AP/FollowCtrl/PlausibilityCheck/Subsystem ==
  velTargRel : Inport
  accelTargAbsEnable : Inport  Port=2
  distDesCur : Inport  Port=3
  velSubj : Inport  Port=4
  distTargRel : Inport  Port=5
  Add : Sum
  Compare To Constant : simulink/Logic and Bit Operations/Compare To Constant  relop=<  const=P_LongCtrl_FollowQuickDecelVelTargRelThres  OutDataTypeStr=boolean
  Compare To Constant3 : simulink/Logic and Bit Operations/Compare To Constant  relop=>  const=P_LongCtrl_FollowQuickDecelVelSubjThres  OutDataTypeStr=boolean
  Compare To Constant4 : simulink/Logic and Bit Operations/Compare To Constant  relop=<  const=P_LongCtrl_FollowQuickAccelTargAbsEnableThres  OutDataTypeStr=boolean
  Constant : Constant  Value=P_LongCtrl_FollowQuickDecelDiffDistRel2DesThres  OutDataTypeStr=single
  Logical Operator : Logic  Inputs=4  AllPortsSameDT=off  OutDataTypeStr=boolean
  Relational Operator : RelationalOperator  Operator=<  OutDataTypeStr=boolean  RndMeth=Simplest
  quickDecel : Outport
  wires:
  velTargRel/1 -> Compare To Constant/1  "velTargRel"
  distTargRel/1 -> Relational Operator/1  "distTargRel"
  distDesCur/1 -> Add/1  "distDesCur"
  velSubj/1 -> Compare To Constant3/1  "velSubj"
  accelTargAbsEnable/1 -> Compare To Constant4/1  "accelTargAbsEnable"
  Add/1 -> Relational Operator/2
  Constant/1 -> Add/2
  Compare To Constant/1 -> Logical Operator/1
  Relational Operator/1 -> Logical Operator/2
  Compare To Constant3/1 -> Logical Operator/3
  Compare To Constant4/1 -> Logical Operator/4
  Logical Operator/1 -> quickDecel/1

== system PvtSubSys_PLAN_AP/AP/AP/FollowCtrl/SlopeStartupAssist/Chart1/coefDistTargRel2AccelCalc ==
  distTargRel : Inport  OutDataTypeStr=single  PortDimensions=1
  distDesCur : Inport  Port=2  OutDataTypeStr=single  PortDimensions=1
  f : TriggerPort  TriggerType=function-call  VariantControl=(inherit)
      settings: CopyFcn=Stateflow.SLINSF.SimulinkMan.removeBlockPreDeleteFcn  PreDeleteFcn=Stateflow.SLINSF.SimulinkMan.unsafePredeleteFcn
  1-D Lookup Table : Lookup_n-D  NumberOfTableDimensions=1  BreakpointsForDimension1=P_LongCtrl_FollowDistDiffCharCoefEnlargeAccelStartUpAssistXAxis  Table=P_LongCtrl_FollowCoefCharDistCoefEnlargeAccelStartUpAssistYAxis  ExtrapMethod=Clip  InternalRulePriority=Speed  RndMeth=Simplest  InputSameDT=on
  Add : Sum  Inputs=+-
  coefDistTargRel2Accel : Outport
  wires:
  distTargRel/1 -> Add/1
  distDesCur/1 -> Add/2
  Add/1 -> 1-D Lookup Table/1
  1-D Lookup Table/1 -> coefDistTargRel2Accel/1

== system PvtSubSys_PLAN_AP/AP/AP/FollowCtrl/SlopeStartupAssist/Chart1/coefVelTargRel2AccelCalc ==
  velTargRel : Inport  OutDataTypeStr=single  PortDimensions=1
  f : TriggerPort  TriggerType=function-call  VariantControl=(inherit)
      settings: CopyFcn=Stateflow.SLINSF.SimulinkMan.removeBlockPreDeleteFcn  PreDeleteFcn=Stateflow.SLINSF.SimulinkMan.unsafePredeleteFcn
  1-D Lookup Table : Lookup_n-D  NumberOfTableDimensions=1  BreakpointsForDimension1=P_LongCtrl_FollowVelCharCoefEnlargeAccelStartUpAssistXAxis  Table=P_LongCtrl_FollowCoefCharVelCoefEnlargeAccelStartUpAssistYAxis  ExtrapMethod=Clip  InternalRulePriority=Speed  RndMeth=Simplest  InputSameDT=on
  coefVelTargRel2Accel : Outport
  wires:
  velTargRel/1 -> 1-D Lookup Table/1
  1-D Lookup Table/1 -> coefVelTargRel2Accel/1

== system PvtSubSys_PLAN_AP/AP/AP/FollowCtrl/VelPlan/Gap ==
  distTargRel : Inport
  velSubj : Inport  Port=2
  Add : Sum  Inputs=+-
  Constant : Constant  Value=0.7  OutDataTypeStr=single
  Constant1 : Constant  Value=0.1  OutDataTypeStr=single
  Constant2 : Constant  Value=4  OutDataTypeStr=single
  MinMax : MinMax  Function=max  Inputs=2
  MinMax1 : MinMax  Inputs=2
  Product : Product  Inputs=*/
  Product1 : Product
  Gap : Outport
  wires:
  Product/1 -> Gap/1
  velSubj/1 -> MinMax/2
  distTargRel/1 -> Product1/1, Add/1
  Add/1 -> Product/1
  MinMax1/1 -> Add/2
  Constant2/1 -> MinMax1/2
  Product1/1 -> MinMax1/1
  Constant/1 -> Product1/2
  MinMax/1 -> Product/2
  Constant1/1 -> MinMax/1

== system PvtSubSys_PLAN_AP/AP/AP/IC/AccelKap/LP ==
  In1 : Inport
  Add5 : Sum  Inputs=+-
  Add6 : Sum
  Constant12 : Constant  Value=0.02  OutDataTypeStr=single
  Constant13 : Constant  Value=0.3  OutDataTypeStr=single
  Product7 : Product  Inputs=*/
  Product8 : Product
  Unit Delay : UnitDelay  SampleTime=-1  HasFrameUpgradeWarning=on
  Out1 : Outport
  wires:
  Constant12/1 -> Product7/1
  Constant13/1 -> Product7/2
  Product7/1 -> Product8/1
  In1/1 -> Add5/1
  Product8/1 -> Add6/1
  Add6/1 -> Out1/1, Unit Delay/1
  Unit Delay/1 -> Add5/2, Add6/2
  Add5/1 -> Product8/2

== system PvtSubSys_PLAN_AP/AP/AP/IC/CurvatureOfMapCalc/Chart/accelICCurvatureMapDistExceed ==
  LongCtrl_IC_EHRV2_CurDisMatrix : Inport  OutDataTypeStr=single  PortDimensions=1
  velDelta : Inport  Port=2  OutDataTypeStr=single  PortDimensions=1
  f : TriggerPort  TriggerType=function-call  VariantControl=(inherit)
      settings: CopyFcn=Stateflow.SLINSF.SimulinkMan.removeBlockPreDeleteFcn  PreDeleteFcn=Stateflow.SLINSF.SimulinkMan.unsafePredeleteFcn
  Constant : Constant  Value=2  OutDataTypeStr=single
  Constant1 : Constant  Value=-1  OutDataTypeStr=single
  Constant2 : Constant  Value=10  OutDataTypeStr=single
  Math Function : Math  Operator=magnitude^2  SaturateOnIntegerOverflow=on
  MinMax : MinMax  Function=max  Inputs=2
  Product : Product
  Product1 : Product  Inputs=*/
  Product2 : Product
  accelICCurvatureMapMatrix : Outport
  wires:
  LongCtrl_IC_EHRV2_CurDisMatrix/1 -> MinMax/1
  Constant/1 -> Product/2
  Product2/1 -> accelICCurvatureMapMatrix/1  "accelICCurvatureMapMatrix"
  velDelta/1 -> Math Function/1
  Math Function/1 -> Product1/1
  Product/1 -> Product1/2
  Product1/1 -> Product2/1
  Constant1/1 -> Product2/2
  Constant2/1 -> MinMax/2
  MinMax/1 -> Product/1

== system PvtSubSys_PLAN_AP/AP/AP/IC/CurvatureOfMapCalc/Chart/accelICCurvatureMapNegCalc ==
  velDelta : Inport  OutDataTypeStr=single  PortDimensions=1
  f : TriggerPort  TriggerType=function-call  VariantControl=(inherit)
      settings: CopyFcn=Stateflow.SLINSF.SimulinkMan.removeBlockPreDeleteFcn  PreDeleteFcn=Stateflow.SLINSF.SimulinkMan.unsafePredeleteFcn
  Constant : Constant  Value=P_LongCtrl_ICtAcceleTimeNegCurvatureMap  OutDataTypeStr=single
  Product : Product  Inputs=*/
  accelICCurvatureMapMatrix : Outport
  wires:
  velDelta/1 -> Product/1
  Constant/1 -> Product/2
  Product/1 -> accelICCurvatureMapMatrix/1  "accelICCurvatureMapMatrix"

== system PvtSubSys_PLAN_AP/AP/AP/IC/CurvatureOfMapCalc/Chart/accelICCurvatureMapPosCalc ==
  velDelta : Inport  OutDataTypeStr=single  PortDimensions=1
  f : TriggerPort  TriggerType=function-call  VariantControl=(inherit)
      settings: CopyFcn=Stateflow.SLINSF.SimulinkMan.removeBlockPreDeleteFcn  PreDeleteFcn=Stateflow.SLINSF.SimulinkMan.unsafePredeleteFcn
  Constant : Constant  Value=P_LongCtrl_ICtAcceleTimePosCurvatureMap  OutDataTypeStr=single
  Product : Product  Inputs=*/
  accelICCurvatureMapMatrix : Outport
  wires:
  velDelta/1 -> Product/1
  Constant/1 -> Product/2
  Product/1 -> accelICCurvatureMapMatrix/1  "accelICCurvatureMapMatrix"

== system PvtSubSys_PLAN_AP/AP/AP/IC/CurvatureOfMapCalc/Chart/distDesCurvatureMapCalc ==
  velDelta : Inport  OutDataTypeStr=single  PortDimensions=1
  accelICCurvatureMapMatrix : Inport  Port=2  OutDataTypeStr=single  PortDimensions=1
  f : TriggerPort  TriggerType=function-call  VariantControl=(inherit)
      settings: CopyFcn=Stateflow.SLINSF.SimulinkMan.removeBlockPreDeleteFcn  PreDeleteFcn=Stateflow.SLINSF.SimulinkMan.unsafePredeleteFcn
  Abs : Abs
  Constant : Constant  Value=2  OutDataTypeStr=single
  Math Function : Math  Operator=magnitude^2  SaturateOnIntegerOverflow=on
  Product : Product  Inputs=*/
  Product1 : Product
  distDesCurvatureMap : Outport
  wires:
  velDelta/1 -> Math Function/1
  Math Function/1 -> Product/1
  accelICCurvatureMapMatrix/1 -> Abs/1
  Constant/1 -> Product1/2
  Product1/1 -> Product/2
  Product/1 -> distDesCurvatureMap/1  "distDesCurvatureMap"
  Abs/1 -> Product1/1

== system PvtSubSys_PLAN_AP/AP/AP/IC/CurvatureOfMapCalc/Chart/velDeltaCalc ==
  velSubjLimMap : Inport  OutDataTypeStr=single  PortDimensions=[1 10]
  velSubj : Inport  Port=2  OutDataTypeStr=single  PortDimensions=1
  f : TriggerPort  TriggerType=function-call  VariantControl=(inherit)
      settings: CopyFcn=Stateflow.SLINSF.SimulinkMan.removeBlockPreDeleteFcn  PreDeleteFcn=Stateflow.SLINSF.SimulinkMan.unsafePredeleteFcn
  Add : Sum  Inputs=+-
  velDelta : Outport
  wires:
  velSubjLimMap/1 -> Add/1
  velSubj/1 -> Add/2
  Add/1 -> velDelta/1  "velDelta"
